simulink model "model_sim"  (R2023b)
settings: Solver=FixedStepAuto  StartTime=0.0  StopTime=tsim  FixedStep=T  RelTol=1e-3
values from neighbouring files (symbols this model uses):
  Kd = [12, 0.15]    [program.m]
  Kp = [4.5, 0.2]    [program.m]
undefined symbols (not defined in the file or in its folder): Ki, T
libraries: slpidlib x2
settings Model: Creator=usuario  LastModifiedBy=usuario
settings DataIOCC: ReturnWorkspaceOutputs=off  TimeSaveName=t

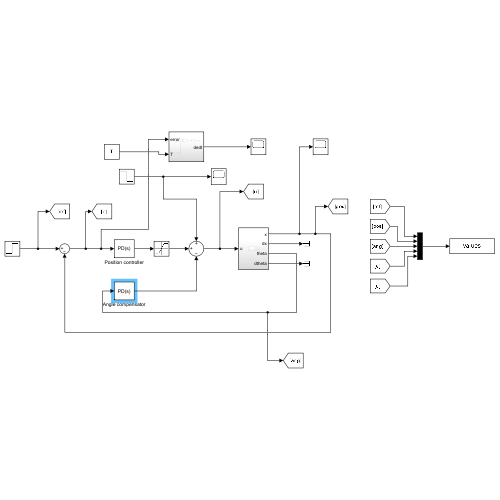
[thumbnail: Simulink's stored preview of the top-level diagram]
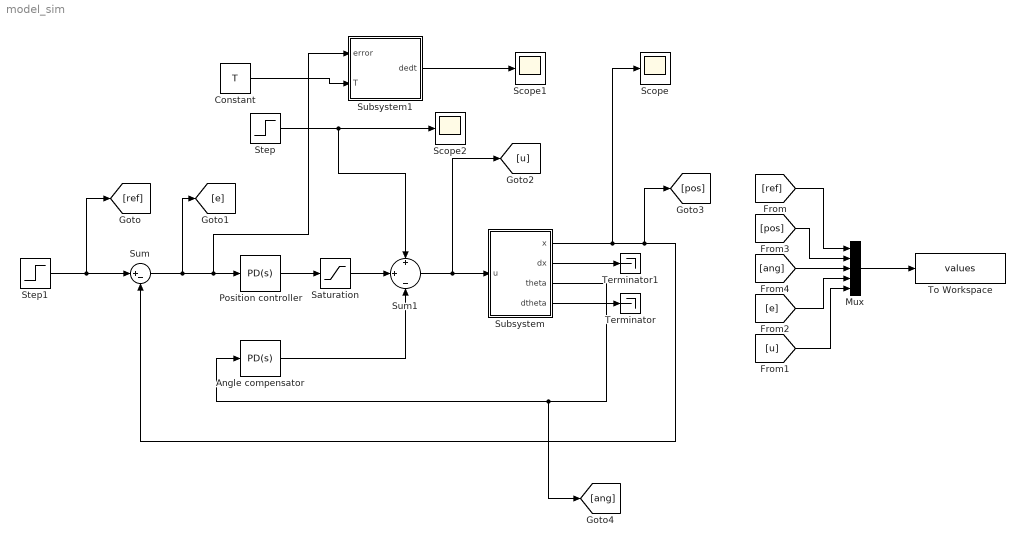
== system model_sim ==
  Angle compensator : slpidlib/PID Controller  Controller=PD  Form=Parallel  TimeDomain=Continuous-time  UseExternalTs=off  SampleTime=-1  IntegratorMethod=Forward Euler  FilterMethod=Forward Euler  ControllerParametersSource=internal  P=Kp(2)  I=1  UseKiTs=off  D=Kd(2)  N=10  UseFilter=on  TunerSelectOption=Transfer Function Based (PID Tuner App)  InitialConditionSource=internal  InitialConditionForIntegrator=0  InitialConditionForFilter=0  DifferentiatorICPrevScaledInput=0  ExternalReset=none  TrackingMode=off  Kt=1  LimitOutput=off  SatLimitsSource=internal  UpperSaturationLimit=inf  LowerSaturationLimit=-inf  LinearizeAsGain=on  AntiWindupMode=none  Kb=1  LimitIntegrator=off  UpperIntegratorSaturationLimit=inf  LowerIntegratorSaturationLimit=-inf  POutMin=[]  POutMax=[]  IOutMin=[]  IOutMax=[]  DOutMin=[]  DOutMax=[]  NOutMin=[]  NOutMax=[]  SumOutMin=[]  SumOutMax=[]  SaturationOutMin=[]  SaturationOutMax=[]  PParamMin=[]  PParamMax=[]  IParamMin=[]  IParamMax=[]  DParamMin=[]  DParamMax=[]  NParamMin=[]  NParamMax=[]  KbParamMin=[]  KbParamMax=[]  KtParamMin=[]  KtParamMax=[]  KbOutMin=[]  KbOutMax=[]  KtOutMin=[]  KtOutMax=[]  IntegratorOutMin=[]  IntegratorOutMax=[]  FilterOutMin=[]  FilterOutMax=[]  SumI1OutMin=[]  SumI1OutMax=[]  SumI2OutMin=[]  SumI2OutMax=[]  SumI3OutMin=[]  SumI3OutMax=[]  SumI4OutMin=[]  SumI4OutMax=[]  SumDOutMin=[]  SumDOutMax=[]  DifferentiatorOutMin=[]  DifferentiatorOutMax=[]  FilterDiffOutCoefMin=[]  FilterDiffOutCoefMax=[]  ReciprocalOutMin=[]  ReciprocalOutMax=[]  SumDenOutMin=[]  SumDenOutMax=[]  SumNumOutMin=[]  SumNumOutMax=[]  DivideOutMin=[]  DivideOutMax=[]  UdiffTsProdOutMin=[]  UdiffTsProdOutMax=[]  NTsProdOutMin=[]  NTsProdOutMax=[]  UintegralTsProdOutMin=[]  UintegralTsProdOutMax=[]  UngainTsProdOutMin=[]  UngainTsProdOutMax=[]  ClampingZeroOutDataTypeStr=Inherit: Inherit via back propagation  ClampingZeroOutMin=[]  ClampingZeroOutMax=[]  FilterDenConstantOutDataTypeStr=Inherit: Inherit via back propagation  FilterDenConstantOutMin=[]  FilterDenConstantOutMax=[]  PCopyOutDataTypeStr=Inherit: Inherit via back propagation  PCopyOutMin=[]  PCopyOutMax=[]  NCopyOutDataTypeStr=Inherit: Inherit via back propagation  NCopyOutMin=[]  NCopyOutMax=[]  IntegratorContinuousStateAttributes=''  IntegratorStateMustResolveToSignalObject=off  IntegratorRTWStateStorageClass=Auto  FilterContinuousStateAttributes=''  FilterStateMustResolveToSignalObject=off  FilterRTWStateStorageClass=Auto  ParallelPVariant=InternalParameters  IdealPVariant=Disabled  IVariant=Disabled  DVariant=InternalParameters  IntegratorVariant=Disabled  SatVariant=Disabled  AWVariant=Disabled  PCopyVariant=Disabled  TRVariant=Disabled  FdbkBlocksVariant=Forward  IdealPFdbkVariant=Disabled  SatFdbkVariant=Disabled  DerivativeFilterVariant=ContFilter  NVariant=InternalParameters  NCopyVariant=Disabled  FilterICVariant=InternalICsFilter  IntegratorICVariant=Disabled  ExternalResetVariant=Disabled  TRSumVariant=Passthrough  SumFdbkVariant=Disabled  SumVariant=Sum_PD  TsampFilterVariant=InternalTs  TsampNgainVariant=Passthrough  TsampIntegralVariant=Disabled_SignalSpec  ExternalSaturationOutDataTypeStr=Inherit: Same as second input
  Constant : Constant  Value=T
  Mux : Mux  Inputs=5
  Position controller : slpidlib/PID Controller  Controller=PD  Form=Parallel  TimeDomain=Continuous-time  UseExternalTs=off  SampleTime=-1  IntegratorMethod=Forward Euler  FilterMethod=Forward Euler  ControllerParametersSource=internal  P=Kp(1)  I=Ki  UseKiTs=off  D=Kd(1)  N=10  UseFilter=on  TunerSelectOption=Transfer Function Based (PID Tuner App)  InitialConditionSource=internal  InitialConditionForIntegrator=0  InitialConditionForFilter=0  DifferentiatorICPrevScaledInput=0  ExternalReset=none  TrackingMode=off  Kt=1  LimitOutput=off  SatLimitsSource=internal  UpperSaturationLimit=inf  LowerSaturationLimit=-inf  LinearizeAsGain=on  AntiWindupMode=none  Kb=1  LimitIntegrator=off  UpperIntegratorSaturationLimit=inf  LowerIntegratorSaturationLimit=-inf  POutMin=[]  POutMax=[]  IOutMin=[]  IOutMax=[]  DOutMin=[]  DOutMax=[]  NOutMin=[]  NOutMax=[]  SumOutMin=[]  SumOutMax=[]  SaturationOutMin=[]  SaturationOutMax=[]  PParamMin=[]  PParamMax=[]  IParamMin=[]  IParamMax=[]  DParamMin=[]  DParamMax=[]  NParamMin=[]  NParamMax=[]  KbParamMin=[]  KbParamMax=[]  KtParamMin=[]  KtParamMax=[]  KbOutMin=[]  KbOutMax=[]  KtOutMin=[]  KtOutMax=[]  IntegratorOutMin=[]  IntegratorOutMax=[]  FilterOutMin=[]  FilterOutMax=[]  SumI1OutMin=[]  SumI1OutMax=[]  SumI2OutMin=[]  SumI2OutMax=[]  SumI3OutMin=[]  SumI3OutMax=[]  SumI4OutMin=[]  SumI4OutMax=[]  SumDOutMin=[]  SumDOutMax=[]  DifferentiatorOutMin=[]  DifferentiatorOutMax=[]  FilterDiffOutCoefMin=[]  FilterDiffOutCoefMax=[]  ReciprocalOutMin=[]  ReciprocalOutMax=[]  SumDenOutMin=[]  SumDenOutMax=[]  SumNumOutMin=[]  SumNumOutMax=[]  DivideOutMin=[]  DivideOutMax=[]  UdiffTsProdOutMin=[]  UdiffTsProdOutMax=[]  NTsProdOutMin=[]  NTsProdOutMax=[]  UintegralTsProdOutMin=[]  UintegralTsProdOutMax=[]  UngainTsProdOutMin=[]  UngainTsProdOutMax=[]  ClampingZeroOutDataTypeStr=Inherit: Inherit via back propagation  ClampingZeroOutMin=[]  ClampingZeroOutMax=[]  FilterDenConstantOutDataTypeStr=Inherit: Inherit via back propagation  FilterDenConstantOutMin=[]  FilterDenConstantOutMax=[]  PCopyOutDataTypeStr=Inherit: Inherit via back propagation  PCopyOutMin=[]  PCopyOutMax=[]  NCopyOutDataTypeStr=Inherit: Inherit via back propagation  NCopyOutMin=[]  NCopyOutMax=[]  IntegratorContinuousStateAttributes=''  IntegratorStateMustResolveToSignalObject=off  IntegratorRTWStateStorageClass=Auto  FilterContinuousStateAttributes=''  FilterStateMustResolveToSignalObject=off  FilterRTWStateStorageClass=Auto  ParallelPVariant=InternalParameters  IdealPVariant=Disabled  IVariant=Disabled  DVariant=InternalParameters  IntegratorVariant=Disabled  SatVariant=Disabled  AWVariant=Disabled  PCopyVariant=Disabled  TRVariant=Disabled  FdbkBlocksVariant=Forward  IdealPFdbkVariant=Disabled  SatFdbkVariant=Disabled  DerivativeFilterVariant=ContFilter  NVariant=InternalParameters  NCopyVariant=Disabled  FilterICVariant=InternalICsFilter  IntegratorICVariant=Disabled  ExternalResetVariant=Disabled  TRSumVariant=Passthrough  SumFdbkVariant=Disabled  SumVariant=Sum_PD  TsampFilterVariant=InternalTs  TsampNgainVariant=Passthrough  TsampIntegralVariant=Disabled_SignalSpec  ExternalSaturationOutDataTypeStr=Inherit: Same as second input
  Saturation : Saturate  UpperLimit=10  LowerLimit=-10
  Scope : Scope
  Scope1 : Scope
  Scope2 : Scope
  Step : Step  Time=10  After=-5  SampleTime=0
  Step1 : Step  After=5  SampleTime=0
  Subsystem : Subsystem
  Subsystem1 : Subsystem
  Sum : Sum  Inputs=|+-
  Sum1 : Sum  Inputs=+|+|-
  Terminator : Terminator
  Terminator1 : Terminator
  To Workspace : ToWorkspace  VariableName=values  SaveFormat=Structure  SampleTime=-1
  wires:
  Mux/1 -> To Workspace/1
  Subsystem/1(x) -> Scope/1, [pos], Sum/2
  Subsystem/3(theta) -> [ang], Angle compensator/1
  Sum/1 -> [e], Subsystem1/1(error), Position controller/1
  Step1/1 -> [ref], Sum/1
  Subsystem/4(dtheta) -> Terminator/1
  Subsystem/2(dx) -> Terminator1/1
  [ref] -> Mux/1
  [pos] -> Mux/2
  [ang] -> Mux/3
  [e] -> Mux/4
  [u] -> Mux/5
  Angle compensator/1 -> Sum1/3
  Step/1 -> Scope2/1, Sum1/1
  Sum1/1 -> [u], Subsystem/1(u)
  Position controller/1 -> Saturation/1
  Saturation/1 -> Sum1/2
  Constant/1 -> Subsystem1/2(T)
  Subsystem1/1(dedt) -> Scope1/1

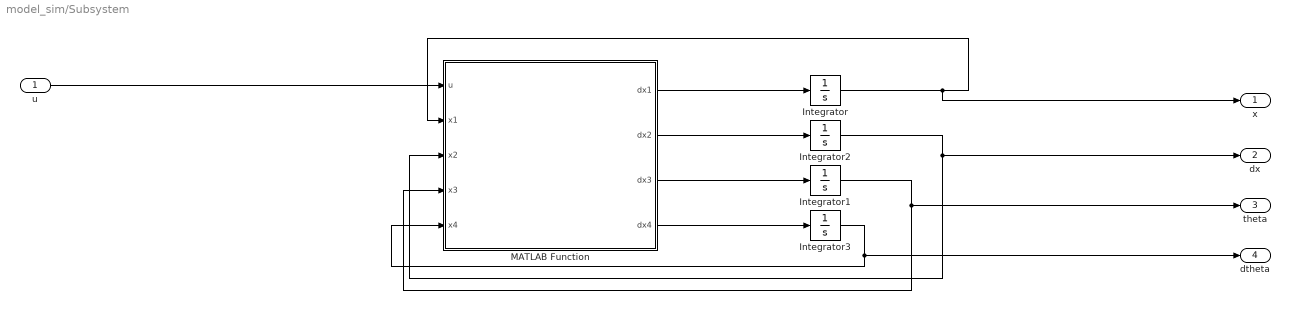
== system model_sim/Subsystem ==
  u : Inport
  Integrator : Integrator  InitialCondition=0.002
  Integrator1 : Integrator  InitialCondition=0.001
  Integrator2 : Integrator
  Integrator3 : Integrator
  MATLAB Function : MATLAB Function  TreatAsAtomicUnit=on
  x : Outport
  dx : Outport  Port=2
  theta : Outport  Port=3
  dtheta : Outport  Port=4
  wires:
  MATLAB Function/2(dx2) -> Integrator2/1
  Integrator/1 -> x/1, MATLAB Function/2(x1)
  Integrator2/1 -> MATLAB Function/3(x2), dx/1
  MATLAB Function/4(dx4) -> Integrator3/1
  MATLAB Function/1(dx1) -> Integrator/1
  MATLAB Function/3(dx3) -> Integrator1/1
  Integrator3/1 -> MATLAB Function/5(x4), dtheta/1
  Integrator1/1 -> theta/1, MATLAB Function/4(x3)
  u/1 -> MATLAB Function/1(u)

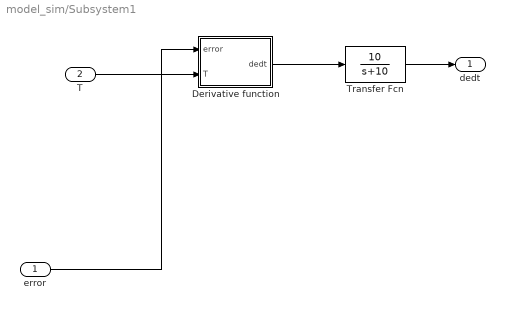
== system model_sim/Subsystem1 ==
  error : Inport
  T : Inport  Port=2
  Derivative function : MATLAB Function  TreatAsAtomicUnit=on  SystemSampleTime=T
  Transfer Fcn : TransferFcn  Numerator=[10]  Denominator=[1 10]
  dedt : Outport
  wires:
  error/1 -> Derivative function/1(error)
  Derivative function/1(dedt) -> Transfer Fcn/1
  T/1 -> Derivative function/2(T)
  Transfer Fcn/1 -> dedt/1

== matlab function model_sim/Subsystem1/Derivative function ==
  data: error input; dedt output; T input
function dedt = fcn(error, T)
    persistent p_error;
    if isempty(p_error)
        p_error = error;
    end
    dedt = (p_error - error)/T;
    p_error = error;
end

== matlab function model_sim/Subsystem/MATLAB Function ==
  data: u input; dx1 output; x1 input; x2 input; x3 input; x4 input; dx2 output; dx3 output; dx4 output
function [dx1,dx2,dx3,dx4] = plant_model(u,x1,x2,x3,x4)
M = 10;g=9.8;m=0.8;l=0.5;mu=0.05;
q = [x1;x2;x3;x4];
a11 = -mu/(M+m*sin(x3)^2); a12 = m*g*cos(x3)*sin(x3)/((M+m*sin(x3)^2)*x3);
a13 = m*l*x4*sin(x3)/(M+m*sin(x3)^2); a21 = mu*cos(x3)/(l*(M+m*sin(x3)^2));
a22 = -(M+m)*g*sin(x3)/(l*x3*(M+m*sin(x3)^2)); a23=-m*x4*sin(x3)*cos(x3)/(M+m*sin(x3)^2);
b1 = 1/(M+m*sin(x3)^2); b2 = -cos(x3)/(l*(M+m*sin(x3)^2));
A = [0 1 0 0;0 a11 a12 a13;0 0 0 1;0 a21 a22 a23];
B = [0;b1;0;b2];

dq = A*q + B*u;
dx1 = dq(1);
dx2 = dq(2);
dx3 = dq(3);
dx4 = dq(4);
